simulink model "Microgrid_with_Utility_Connection"  (R2024b)
settings: Solver=daessc  StartTime=0.0  StopTime=inf  MaxStep=1e-3  RelTol=1e-3  AbsTol=1e-3
values from neighbouring files (symbols this model uses):
  Bat =     [initData.mat]
  droopFC1 = 0.05    [initData.mat]
  droopFC2 = 0.05    [initData.mat]
  droopP2 = 0.05    [initData.mat]
  droopQ1 = 0.05    [initData.mat]
  droopQ2 = 0.05    [initData.mat]
  Pref2 = 0.8    [initData.mat]
  Qref1 = 0    [initData.mat]
  Qref2 = 0    [initData.mat]
  timeACLoadCurtail = 200    [initData.mat]
  timeSolarCurtail = 200    [initData.mat]
  Ts = 5e-05    [initData.mat]
  Ts_AC = 0.0002    [initData.mat]
  Ts_DC = 0.001    [initData.mat]
  volt2 = [270.467186401 250.166401688 246.278575679 243.847178474 242.073246789 240.654489675 239.457734124 238.414696845 237.485238449 236.643553985 235.871256975 235.151075236 ... (161 elements, 1x161)]    [initData.mat]
undefined symbols (not defined in the file or in its folder): BattTempBp, CapLUTBp, CapSOCBp, DiscIntNeverNeededParam, Em, Np, Ns, RInt, Tc_Batt
libraries: nesl_utility x62, fl_lib x55, ee_lib x41, modbuslib x16, spsRMSLib x8, simulink x5, spsFourierLib x2, batteryecm_lib x1, eeTransforms x1
(part 2 of 3)

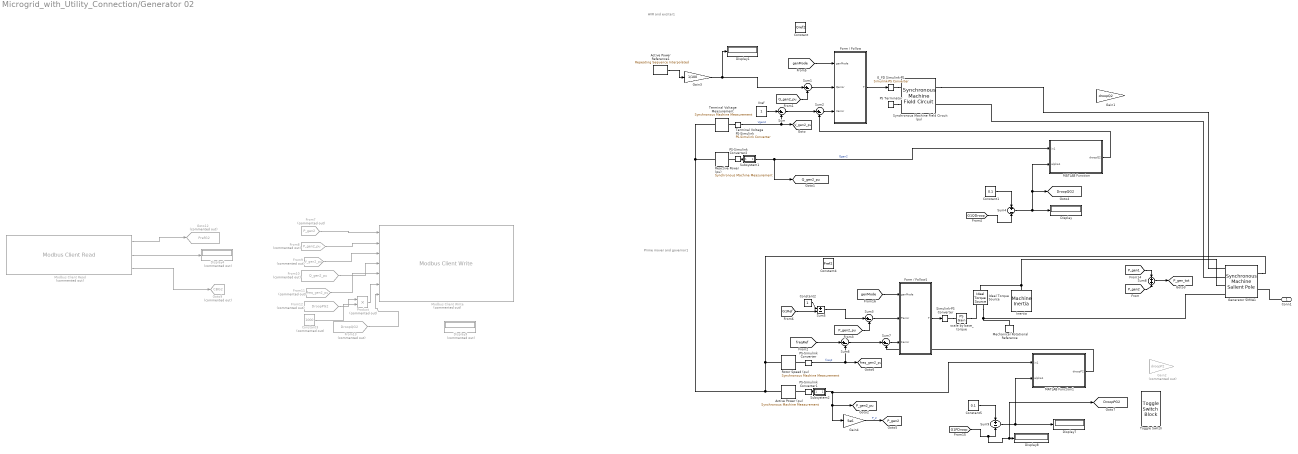
== system Microgrid_with_Utility_Connection/Generator 02 ==
  note: Prime mover
      | and governor1
  note: AVR and exciter1
  "Active Power (pu) " : ee_lib/Electromechanical/Synchronous/Synchronous Machine Measurement  output_idx=12
      settings: InternalSimscapePortConfiguration="{\"Bottom\":[],\"Left\":[{\"id\":\"pu_input\",\"label\":\"pu\",\"type\":\"input\"}],\"Right\":[{\"id\":\"pu_output\",\"label\":\"o\",\"type\":\"output\"}],\"Top\":[]}"
  Active Power Reference1 : simulink/Sources/Repeating Sequence Interpolated  OutValues=[0 0 0 0 0 0]  TimeValues=[100 110 120 130 140 500]  LookUpMeth=Interpolation-Use End Values  tsamp=Ts_AC  OutMin=[]  OutMax=[]  OutDataTypeStr=double  OutputDataTypeScalingMode=double  OutDataType=fixdt(0,8)  OutScaling=2^-10
  Constant : Constant  Value=Qref2
  Constant1 : Constant  Value=0.1
  Constant2 : Constant
  Constant3 : Constant  Commented=on  Value=1000
  Constant4 : Constant  Value=Pref2
  Constant5 : Constant  Value=0.1
  Display{,1,7..8} (4 alike) : Display
  Display4 : Display  Commented=on
      settings: Format=decimal (Stored Integer)  Decimation=4
  Display9 : Display  Commented=on
  "E_FD Simulink-PS " : nesl_utility/Simulink-PS Converter  PhysicalDomain=network_engine_domain  SubClassName=ps_input  LeftPortType=input  RightPortType=output  PseudoPeriodic=off  Frequencies=[]  NoiseDistribution=none  NoiseParameters=[]  Unit=1  AffineConversion=off  FilteringAndDerivatives=provide  SimscapeFilterOrder=1  InputFilterTimeConstant=.001  UdotUserProvided=0
  Form / Follow : Subsystem
  Form / Follow1 : Subsystem
  From10 : From  Commented=on  GotoTag=Q_gen2_pu  TagVisibility=global
  From11 : From  Commented=on  GotoTag=freq_gen2_pu  TagVisibility=global
  From12 : From  Commented=on  GotoTag=DroopPG2  TagVisibility=global
  From13 : From  Commented=on  GotoTag=DroopQG2  TagVisibility=global
  From7 : From  Commented=on  GotoTag=P_gen2  TagVisibility=global
  From8 : From  Commented=on  GotoTag=P_gen2_pu  TagVisibility=global
  From9 : From  Commented=on  GotoTag=V_gen2_pu  TagVisibility=global
  Gain1 : Gain  Gain=droopQ2
  Gain2 : Gain  Commented=on  Gain=droopP2
  Gain3 : Gain  Gain=1/100
  Gain4 : Gain  Gain=5e6
  Generator 5MVA1 : ee_lib/Electromechanical/Synchronous/Synchronous Machine Salient Pole  port_option=ee.enum.threePhasePort.composite  SRated=5e6 A*V  VRated=6600 V  FRated=50 Hz  nPolePairs=4  param_option=ee.enum.sm.parameterization.standard  fieldCircuitParameterization_option=ee.enum.sm.fieldparameterization.current  baseEfd=216.54 V  baseIfd=50 A  zero_sequence=ee.enum.park.zerosequence.exclude  axes_param=ee.enum.rotorangle.daxis  Ladu=0.9  Laqu=0.55  L0=0.15  Ll=0.15  Ra=0.011  Lfd=0.2571  Rfd=0.0006  L1d=0.2  R1d=0.0354  L1q=0.2567  R1q=0.0428  Xl=0.15  Xd=1.05  Xq=0.7  X0=0.15  Xdd=0.35  Xddd=0.25  Xqdd=0.325  d_option=ee.enum.circuit.open  Td0d=5.25 s  Tdd=1.75 s  Td0dd=0.03 s  Tddd=0.0214 s  q_option=ee.enum.circuit.open  Tq0dd=0.05 s  Tqdd=0.0232 s  saturation_option=ee.enum.saturation.exclude  saturation_ifd=[0.00, 0.48, 0.76, 1.38, 1.79]  saturation_Vag=[0.00, 0.43, 0.59, 0.71, 0.76]  initialization_option=ee.enum.sm.initialization.electrical  source_type=ee.enum.sm.load_flow_source_type.Swing  Vmag0=6600 V  Vang0=0 deg  Pt0=0.5 A*V  Qt0=0 A*V  minimum_pu=0.95  phase_search_range=[-inf, inf] deg  gmin=1e-6 S  connection_option=ee.enum.Connection.wye  num_q_dampers=1  rotor_offset=-pi / 2 rad  pu_psid_specify=on  pu_psid_priority=High  pu_psid=0  pu_psid_nominal_specify=off  pu_psid_nominal_value=1  pu_psid_nominal_unit=1  pu_psiq_specify=on  pu_psiq_priority=High  pu_psiq=0  pu_psiq_nominal_specify=off  pu_psiq_nominal_value=1  pu_psiq_nominal_unit=1  pu_psifd_specify=on  pu_psifd_priority=High  pu_psifd=0  pu_psifd_nominal_specify=off  pu_psifd_nominal_value=1  pu_psifd_nominal_unit=1  pu_psi1d_specify=on  pu_psi1d_priority=High  pu_psi1d=0  pu_psi1d_nominal_specify=off  pu_psi1d_nominal_value=1  pu_psi1d_nominal_unit=1  pu_psi1q_specify=on  pu_psi1q_priority=High  pu_psi1q=0  pu_psi1q_nominal_specify=off  pu_psi1q_nominal_value=1  pu_psi1q_nominal_unit=1  angular_position_diff_specify=on  angular_position_diff_priority=High  angular_position_diff=0 deg  angular_position_diff_nominal_specify=off  angular_position_diff_nominal_value=1  angular_position_diff_nominal_unit=deg  Tmeas=298.15 K  alpha=3.93e-3 1/K  stator_thermal_mass=100 J/K  rotor_thermal_mass=200 J/K  temperatureA_specify=off  temperatureA_priority=High  temperatureA=25 degC  temperatureA_nominal_specify=off  temperatureA_nominal_value=1  temperatureA_nominal_unit=degC  temperatureB_specify=off  temperatureB_priority=High  temperatureB=25 degC  temperatureB_nominal_specify=off  temperatureB_nominal_value=1  temperatureB_nominal_unit=degC  temperatureC_specify=off  temperatureC_priority=High  temperatureC=25 degC  temperatureC_nominal_specify=off  temperatureC_nominal_value=1  temperatureC_nominal_unit=degC  temperatureR_specify=off  temperatureR_priority=High  temperatureR=25 degC  temperatureR_nominal_specify=off  temperatureR_nominal_value=1  temperatureR_nominal_unit=degC
      settings: LogSimulationData=on  InternalSimscapePortConfiguration="{\"Bottom\":[],\"Left\":[{\"id\":\"fd_p\",\"label\":\"fd+\",\"type\":\"foundation.electrical.electrical\"},{\"id\":\"fd_n\",\"label\":\"fd-\",\"type\":\"foundation.electrical.electrical\"},{\"id\":\"R\",\"label\":\"R\",\"type\":\"foundation.mechanical.rotational.rotational\"},{\"id\":\"C\",\"label\":\"C\",\"type\":\"foundation.mechanical.rotational.rotational\"}],\"Right\":[{\"id\":\"pu_output\",\"label\":\"pu\",\"type\":\"output\"},{\"id\":\"N\",\"label\":\"~\",\"type\":\"foundation.electrical.three_phase\"}],\"Top\":[]}"
  Goto12 : Goto  Commented=on  GotoTag=PrefG2  TagVisibility=global
  Goto9 : Goto  Commented=on  GotoTag=CBG2  TagVisibility=global
  Ideal Torque Source : fl_lib/Mechanical/Mechanical Sources/Ideal Torque Source
  Inertia : ee_lib/Electromechanical/Mechanical/Machine Inertia  SRated=5e6 V*A  FRated=50 Hz  nPolePairs=4  inertia_option=2  J=27548 kg*m^2  H=3.525 s*W/V/A  damper_option=2  D=39.0509 N*m/(rad/s)  pu_D=0.01  initialization_option=2  fMechanical0=50 Hz  fElectrical0=50 Hz
      settings: LogSimulationData=on  InternalSimscapePortConfiguration="{\"Bottom\":[],\"Left\":[{\"id\":\"R\",\"label\":\"R\",\"type\":\"foundation.mechanical.rotational.rotational\"}],\"Right\":[],\"Top\":[]}"
  MATLAB Function : MATLAB Function  TreatAsAtomicUnit=on
  MATLAB Function1 : MATLAB Function  TreatAsAtomicUnit=on
  Mechanical Rotational Reference : fl_lib/Mechanical/Rotational Elements/Mechanical Rotational Reference
  Modbus Client Read : modbuslib/Modbus Client Read  Commented=on  RetainClient=gen2  ClientList=gen2  ConnectionEndpoint=192.168.1.203:502  ServerId=1  RegisterTable={ '1', 'PrefG2', '21', 'Holding Register', 'double', '1'; '2', 'QrefG2', '29', 'Holding Register', 'double', '1'; '3', 'CBG2', '38', 'Coil', 'bit', '1' }  SampleTime=1
  Modbus Client Write : modbuslib/Modbus Client Write  Commented=on  RetainClient=gen2  ClientList=gen2  ConnectionEndpoint=192.168.1.203:502  ServerId=1  RegisterTable={ '1', 'P_gen2', '1', 'Holding Register', 'double'; '2', 'P_gen2_pu', '5', 'Holding Register', 'double'; '3', 'V_gen2_pu', '9', 'Holding Register', 'double'; '4', 'Q_gen2_pu', '13', 'Holding Register', 'double'; '5', 'freq_gen2_pu', '17', 'Holding Register', 'double'; '6', 'DroopPG2', '25', 'Holding Register', 'double'; '7', 'DroopQG2', '34', 'Holding Register', 'double' }  SampleTime=1
  PS Terminator : fl_lib/Physical Signals/Sinks/PS Terminator
  PS-Simulink Converter : nesl_utility/PS-Simulink Converter  PhysicalDomain=network_engine_domain  SubClassName=ps_output  LeftPortType=input  RightPortType=output  PseudoPeriodic=off  Frequencies=[]  VectorFormat=1-D array  Unit=inherit  AffineConversion=off
  PS-Simulink Converter1 : nesl_utility/PS-Simulink Converter  PhysicalDomain=network_engine_domain  SubClassName=ps_output  LeftPortType=input  RightPortType=output  PseudoPeriodic=off  Frequencies=[]  VectorFormat=1-D array  Unit=inherit  AffineConversion=off
  PS-Simulink Converter2 : nesl_utility/PS-Simulink Converter  PhysicalDomain=network_engine_domain  SubClassName=ps_output  LeftPortType=input  RightPortType=output  PseudoPeriodic=off  Frequencies=[]  VectorFormat=1-D array  Unit=inherit  AffineConversion=off
  Product : Product  Commented=on
  Reactive Power (pu) : ee_lib/Electromechanical/Synchronous/Synchronous Machine Measurement  output_idx=13
      settings: InternalSimscapePortConfiguration="{\"Bottom\":[],\"Left\":[{\"id\":\"pu_input\",\"label\":\"pu\",\"type\":\"input\"}],\"Right\":[{\"id\":\"pu_output\",\"label\":\"o\",\"type\":\"output\"}],\"Top\":[]}"
  Rotor Speed (pu) : ee_lib/Electromechanical/Synchronous/Synchronous Machine Measurement  output_idx=4
      settings: InternalSimscapePortConfiguration="{\"Bottom\":[],\"Left\":[{\"id\":\"pu_input\",\"label\":\"pu\",\"type\":\"input\"}],\"Right\":[{\"id\":\"pu_output\",\"label\":\"o\",\"type\":\"output\"}],\"Top\":[]}"
  Simulink-PS Converter : nesl_utility/Simulink-PS Converter  PhysicalDomain=network_engine_domain  SubClassName=ps_input  LeftPortType=input  RightPortType=output  PseudoPeriodic=off  Frequencies=[]  NoiseDistribution=none  NoiseParameters=[]  Unit=1  AffineConversion=off  FilteringAndDerivatives=provide  SimscapeFilterOrder=1  InputFilterTimeConstant=0.001  UdotUserProvided=0
  Subsystem1 : Subsystem
  Subsystem2 : Subsystem
  Sum{,1..3,6..7} (6 alike) : Sum  Inputs=|+-
  Sum4 : Sum  Inputs=+-
  Sum5 : Sum  Inputs=+-
  Sum8 : Sum
  Sum9 : Sum  Inputs=+-
  Synchronous Machine Field Circuit (pu) : ee_lib/Electromechanical/Synchronous/Synchronous Machine Field Circuit  unit_option=ee.enum.unit.pu  SRated=5e6 V*A  FRated=50 Hz  fieldCircuitParameterization_option=2  baseEfd=92.95 V  baseIfd=50 A  parameterization_option=2  Ladu=1.66  Rfd=0.0006  Xl=0.15  Xd=1.05  Xdd=0.35  Xddd=0.23  d_option=ee.enum.circuit.open  Td0d=5.25 s  Tdd=1.3260 s  Td0dd=0.03 s  Tddd=0.0230 s
      settings: LogSimulationData=on  InternalSimscapePortConfiguration="{\"Bottom\":[],\"Left\":[{\"id\":\"Efd_pu\",\"label\":\"Efd_pu\",\"type\":\"input\"},{\"id\":\"Ifd_pu\",\"label\":\"Ifd_pu\",\"type\":\"output\"}],\"Right\":[{\"id\":\"fd_p\",\"label\":\"fd+\",\"type\":\"foundation.electrical.electrical\"},{\"id\":\"fd_n\",\"label\":\"fd-\",\"type\":\"foundation.electrical.electrical\"}],\"Top\":[]}"
  Terminal Voltage Measurement : ee_lib/Electromechanical/Synchronous/Synchronous Machine Measurement  output_idx=14
      settings: LogSimulationData=on  InternalSimscapePortConfiguration="{\"Bottom\":[],\"Left\":[{\"id\":\"pu_input\",\"label\":\"pu\",\"type\":\"input\"}],\"Right\":[{\"id\":\"pu_output\",\"label\":\"o\",\"type\":\"output\"}],\"Top\":[]}"
  Terminal Voltage PS-Simulink : nesl_utility/PS-Simulink Converter  PhysicalDomain=network_engine_domain  SubClassName=ps_output  LeftPortType=input  RightPortType=output  PseudoPeriodic=off  Frequencies=[]  VectorFormat=1-D array  Unit=1  AffineConversion=off
  Toggle Switch : ToggleSwitchBlock
      settings: Values={{'Off', 'On'}, [0 0.05]}
  Vref : Constant  SampleTime=Ts_AC
  scale by base_torque : fl_lib/Physical Signals/Functions/PS Gain  gain=53051.6 N*m
  Conn1 : PMIOPort  Side=Right
  tag scope: DroopPG2=global, DroopQG2=global, P_gen2=global, P_gen2_pu=global, P_gen_tot=global, Q_gen2_pu=global, V_gen2_pu=global, freq_gen2_pu=global
  wires:
  Gain3/1 -> Sum1/1, Display1/1
  Active Power Reference1/1 -> Gain3/1
  MATLAB Function/1(droopQ2) -> Sum2/2
  [G1QDroop] -> Sum4/2
  Constant1/1 -> Sum4/1
  Sum4/1 -> [DroopQG2], MATLAB Function/2(alpha1), Display/1
  Form / Follow/1(T) -> "E_FD Simulink-PS "/1
  Sum2/1 -> Form / Follow/3(Verror)
  [genMode] -> Form / Follow/1(genMode)
  Sum1/1 -> Form / Follow/2(Qerror)
  [Q_gen2_pu] -> Sum1/2
  Subsystem1/1(in1) -> MATLAB Function/1(in1), [Q_gen2_pu]  "Qgen2"
  Vref/1 -> Sum/1
  Sum/1 -> Sum2/1
  Terminal Voltage PS-Simulink/1 -> [V_gen2_pu], Sum/2  "Vgen2"
  PS-Simulink Converter2/1 -> Subsystem1/1(In1)
  Constant3/1 -> Product/2
  Product/1 -> Modbus Client Write/6
  From12/1 -> Product/1
  From13/1 -> Modbus Client Write/7
  From11/1 -> Modbus Client Write/5
  From10/1 -> Modbus Client Write/4
  From9/1 -> Modbus Client Write/3
  From8/1 -> Modbus Client Write/2
  Modbus Client Read/3 -> Goto9/1
  From7/1 -> Modbus Client Write/1
  Modbus Client Read/2 -> Display4/1
  Sum5/1 -> Sum3/1
  [G1Ref] -> Sum5/2
  Constant2/1 -> Sum5/1
  [G1PDroop] -> [DroopPG2], Display8/1, Sum9/2
  Constant5/1 -> Sum9/1
  Sum9/1 -> MATLAB Function1/2(alpha1), Display7/1
  Subsystem2/1(in) -> MATLAB Function1/1(in1), [P_gen2_pu], Gain4/1
  Form / Follow1/1(T) -> Simulink-PS Converter/1
  Sum7/1 -> Form / Follow1/3(Ferror)
  Sum3/1 -> Form / Follow1/2(Perror)
  [genMode] -> Form / Follow1/1(genMode)
  [P_gen2_pu] -> Sum3/2
  Sum8/1 -> [P_gen_tot]
  [P_gen2] -> Sum8/2
  [P_gen1] -> Sum8/1
  Gain4/1 -> [P_gen2]  "P_2"
  PS-Simulink Converter1/1 -> Subsystem2/1(In1)
  PS-Simulink Converter/1 -> [freq_gen2_pu], Sum6/2  "freq2"
  [freqRef] -> Sum6/1
  Sum6/1 -> Sum7/1
  MATLAB Function1/1(droopP2) -> Sum7/2
  Modbus Client Read/1 -> Goto12/1
  connections:
  Ideal Torque Source/RConn2 -- Mechanical Rotational Reference/LConn1 -- Generator 5MVA1/LConn4
  Inertia/LConn1 -- Generator 5MVA1/LConn3 -- Ideal Torque Source/LConn1
  Conn1/RConn1 -- Generator 5MVA1/RConn2
  Synchronous Machine Field Circuit (pu)/RConn1 -- Generator 5MVA1/LConn1
  Generator 5MVA1/LConn2 -- Synchronous Machine Field Circuit (pu)/RConn2
  PS Terminator/LConn1 -- Synchronous Machine Field Circuit (pu)/LConn2
  "E_FD Simulink-PS "/RConn1 -- Synchronous Machine Field Circuit (pu)/LConn1
  "Active Power (pu) "/LConn1 -- Reactive Power (pu)/LConn1 -- Terminal Voltage Measurement/LConn1 -- Generator 5MVA1/RConn1 -- Rotor Speed (pu)/LConn1
  Terminal Voltage Measurement/RConn1 -- Terminal Voltage PS-Simulink/LConn1
  PS-Simulink Converter2/LConn1 -- Reactive Power (pu)/RConn1
  Simulink-PS Converter/RConn1 -- scale by base_torque/LConn1
  scale by base_torque/RConn1 -- Ideal Torque Source/RConn1
  PS-Simulink Converter/LConn1 -- Rotor Speed (pu)/RConn1
  PS-Simulink Converter1/LConn1 -- "Active Power (pu) "/RConn1

== system Microgrid_with_Utility_Connection/Grid Synchronization ==
  note: breaker command: 1 - islanded (PCC open)
      | 0 - connect to utility (PCC closed)
  note: 1 - start sycnhronisation
      | 0 - stay islanded
  note: microgrid frequency (pu)
  note: utility grid phase angle
  note: microgrid phase angle
  note: new frequency reference sent to
      | microgrid governer
  note: utility grid frequency (pu)
  note: frequency step size (how aggressive we tune frequency)
  Constant1 : Constant  Value=1e-5
  Constant2 : Constant
  Grid Synchronization1 : MATLAB Function  TreatAsAtomicUnit=on
  Unit Delay : UnitDelay  InitialCondition=1  SampleTime=Ts_AC  HasFrameUpgradeWarning=on
  Unit Delay1 : UnitDelay  InitialCondition=1  SampleTime=Ts_AC  HasFrameUpgradeWarning=on
  tag scope: freqRef=global, gridEnable=global
  wires:
  Grid Synchronization1/2(gridEnable) -> Unit Delay/1  "gridEnable"
  Constant1/1 -> Grid Synchronization1/1(deltaF)
  [phiMicro] -> Grid Synchronization1/5(phiMicro)
  Unit Delay1/1 -> [freqRef]
  [freq_gen1_pu] -> Grid Synchronization1/3(freqMicro)
  Grid Synchronization1/1(freqRef) -> Unit Delay1/1
  Constant2/1 -> Grid Synchronization1/2(freqUtility)
  Unit Delay/1 -> [gridEnable]
  [phiUtility] -> Grid Synchronization1/4(phiUtility)
  [synchStart] -> Grid Synchronization1/6(synchStart)

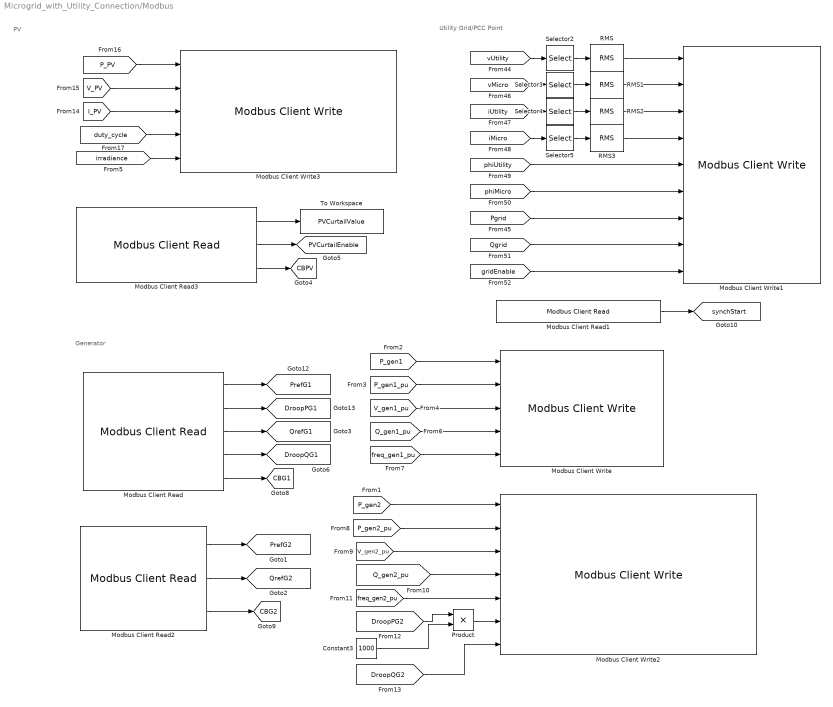
== system Microgrid_with_Utility_Connection/Modbus ==
  note: PV
  note: Utility Grid/PCC Point
  note: Generator
  Constant3 : Constant  Value=1000
  Modbus Client Read : modbuslib/Modbus Client Read  RetainClient=gen1  ClientList=gen1  ConnectionEndpoint=192.168.1.202:502  ServerId=1  RegisterTable={ '1', 'PrefG1', '21', 'Holding Register', 'double', '1'; '2', 'DroopPG1', '25', 'Holding Register', 'double', '1'; '3', 'QrefG1', '29', 'Holding Register', 'double', '1'; '4', 'DroopQG1', '34', 'Holding Register', 'double', '1'; '5', 'CBG1', '38', 'Coil', 'bit', '1' }  SampleTime=1
  Modbus Client Read1 : modbuslib/Modbus Client Read  RetainClient=ModbusClient  ClientList=ModbusClient  ConnectionEndpoint=192.168.1.201:502  ServerId=1  RegisterTable={ '1', 'synchStart', '38', 'Coil', 'bit', '1' }  SampleTime=1
  Modbus Client Read2 : modbuslib/Modbus Client Read  RetainClient=gen2  ClientList=gen2  ConnectionEndpoint=192.168.1.203:502  ServerId=1  RegisterTable={ '1', 'PrefG2', '21', 'Holding Register', 'double', '1'; '2', 'QrefG2', '29', 'Holding Register', 'double', '1'; '3', 'CBG2', '38', 'Coil', 'bit', '1' }  SampleTime=1
  Modbus Client Read3 : modbuslib/Modbus Client Read  RetainClient=pv  ClientList=pv  ConnectionEndpoint=192.168.1.204:502  ServerId=1  RegisterTable={ '1', 'PvCurtailValue', '21', 'Holding Register', 'double', '1'; '2', 'curtail enable', '25', 'Coil', 'bit', '1'; '3', 'CBPV', '29', 'Coil', 'bit', '1' }  SampleTime=1
  Modbus Client Write : modbuslib/Modbus Client Write  RetainClient=gen1  ClientList=gen1  ConnectionEndpoint=192.168.1.202:502  ServerId=1  RegisterTable={ '1', 'P_gen1', '1', 'Holding Register', 'double'; '2', 'P_gen1_pu', '5', 'Holding Register', 'double'; '3', 'V_gen1_pu', '9', 'Holding Register', 'double'; '4', 'Q_gen1_pu', '13', 'Holding Register', 'double'; '5', 'freq_gen1_pu', '17', 'Holding Register', 'double' }  SampleTime=1
  Modbus Client Write1 : modbuslib/Modbus Client Write  RetainClient=ModbusClient  ClientList=ModbusClient  ConnectionEndpoint=192.168.1.201:502  ServerId=1  RegisterTable={ '1', 'vUtility_rms', '1', 'Holding Register', 'double'; '2', 'vMicro_rms', '5', 'Holding Register', 'double'; '3', 'iUtility_rms', '9', 'Holding Register', 'double'; '4', 'iMicro_rms', '13', 'Holding Register', 'double'; '5', 'phiUtility', '17', 'Holding Register', 'double'; '6', 'phiMicro', '21', 'Holding Register', 'double'; '7', 'Pgrid', '25', 'Holding Register', 'double'; '8', 'Qgrid', '29', 'Holding Register', 'double'; '9', 'gridEnable', '34', 'Coil', 'bit' }  SampleTime=1
  Modbus Client Write2 : modbuslib/Modbus Client Write  RetainClient=gen2  ClientList=gen2  ConnectionEndpoint=192.168.1.203:502  ServerId=1  RegisterTable={ '1', 'P_gen2', '1', 'Holding Register', 'double'; '2', 'P_gen2_pu', '5', 'Holding Register', 'double'; '3', 'V_gen2_pu', '9', 'Holding Register', 'double'; '4', 'Q_gen2_pu', '13', 'Holding Register', 'double'; '5', 'freq_gen2_pu', '17', 'Holding Register', 'double'; '6', 'DroopPG2', '25', 'Holding Register', 'double'; '7', 'DroopQG2', '34', 'Holding Register', 'double' }  SampleTime=1
  Modbus Client Write3 : modbuslib/Modbus Client Write  RetainClient=pv  ClientList=pv  ConnectionEndpoint=192.168.1.204:502  ServerId=1  RegisterTable={ '1', 'P_PV', '1', 'Holding Register', 'double'; '2', 'V_PV', '5', 'Holding Register', 'double'; '3', 'I_PV', '9', 'Holding Register', 'double'; '4', 'duty cycle', '13', 'Holding Register', 'double'; '5', 'irradiance', '17', 'Holding Register', 'double' }  SampleTime=1
  Product : Product
  RMS{,1..3} (4 alike) : spsRMSLib/RMS  TrueRMS=on  Freq=50  RMSInit=120  Ts=0
  Selector{2..5} (4 alike) : Selector  InputPortWidth=3  IndexOptions=Index vector (dialog)  Indices=1  OutputSizes=1
  To Workspace : ToWorkspace  VariableName=PVCurtailValue  SaveFormat=Timeseries  SampleTime=-1
  tag scope: CBG1=global, CBG2=global, CBPV=global, DroopPG1=global, DroopQG1=global, PVCurtailEnable=global, PrefG1=global, PrefG2=global, QrefG1=global, QrefG2=global, synchStart=global
  wires:
  [V_gen1_pu] -> Modbus Client Write/3
  [P_gen1_pu] -> Modbus Client Write/2
  Modbus Client Read/1 -> [PrefG1]
  [P_gen1] -> Modbus Client Write/1
  [freq_gen1_pu] -> Modbus Client Write/5
  [Q_gen1_pu] -> Modbus Client Write/4
  Modbus Client Read/2 -> [DroopPG1]
  Modbus Client Read/5 -> [CBG1]
  [iMicro] -> Selector5/1
  RMS2/1 -> Modbus Client Write1/3
  RMS/1 -> Modbus Client Write1/1
  RMS3/1 -> Modbus Client Write1/4
  [iUtility] -> Selector4/1
  [phiUtility] -> Modbus Client Write1/5
  [Qgrid] -> Modbus Client Write1/8
  [Pgrid] -> Modbus Client Write1/7
  Selector4/1 -> RMS2/1
  Selector5/1 -> RMS3/1
  RMS1/1 -> Modbus Client Write1/2
  Modbus Client Read1/1 -> [synchStart]
  [vMicro] -> Selector3/1
  [vUtility] -> Selector2/1
  [phiMicro] -> Modbus Client Write1/6
  [gridEnable] -> Modbus Client Write1/9
  Selector2/1 -> RMS/1
  Selector3/1 -> RMS1/1
  Constant3/1 -> Product/2
  [P_gen2] -> Modbus Client Write2/1
  [DroopPG2] -> Product/1
  [V_gen2_pu] -> Modbus Client Write2/3
  Product/1 -> Modbus Client Write2/6
  Modbus Client Read2/3 -> [CBG2]
  Modbus Client Read2/2 -> [QrefG2]
  [DroopQG2] -> Modbus Client Write2/7
  [freq_gen2_pu] -> Modbus Client Write2/5
  [Q_gen2_pu] -> Modbus Client Write2/4
  [P_gen2_pu] -> Modbus Client Write2/2
  Modbus Client Read2/1 -> [PrefG2]
  Modbus Client Read3/3 -> [CBPV]
  [P_PV] -> Modbus Client Write3/1
  Modbus Client Read3/1 -> To Workspace/1
  [irradiance] -> Modbus Client Write3/5
  [duty_cycle] -> Modbus Client Write3/4
  [I_PV] -> Modbus Client Write3/3
  Modbus Client Read3/2 -> [PVCurtailEnable]
  [V_PV] -> Modbus Client Write3/2
  Modbus Client Read/3 -> [QrefG1]
  Modbus Client Read/4 -> [DroopQG1]

== system Microgrid_with_Utility_Connection/PQ meas ==
  PS-Simulink Converter : nesl_utility/PS-Simulink Converter  PhysicalDomain=network_engine_domain  SubClassName=ps_output  LeftPortType=input  RightPortType=output  PseudoPeriodic=off  Frequencies=[]  VectorFormat=1-D array  Unit=W  AffineConversion=off
  PS-Simulink Converter1 : nesl_utility/PS-Simulink Converter  PhysicalDomain=network_engine_domain  SubClassName=ps_output  LeftPortType=input  RightPortType=output  PseudoPeriodic=off  Frequencies=[]  VectorFormat=1-D array  Unit=V*A  AffineConversion=off
  Power Sensor (Three-Phase) : ee_lib/Sensors & Transducers/Power Sensor (Three-Phase)  load_type=ee.enum.passive.type_balanced.balanced  f0=50 Hz
      settings: InternalSimscapePortConfiguration="{\"Bottom\":[],\"Left\":[{\"id\":\"N1\",\"label\":\"~1\",\"type\":\"foundation.electrical.three_phase\"}],\"Right\":[{\"id\":\"N2\",\"label\":\"~2\",\"type\":\"foundation.electrical.three_phase\"}],\"Top\":[{\"id\":\"Pm\",\"label\":\"P\",\"type\":\"output\"},{\"id\":\"Qm\",\"label\":\"Q\",\"type\":\"output\"}]}"
  Subsystem : Subsystem
  Subsystem1 : Subsystem
  ~1 : PMIOPort  Side=Left
  ~2 : PMIOPort  Port=2  Side=Right
  tag scope: P_load=global, Q_load=global
  wires:
  PS-Simulink Converter1/1 -> Subsystem1/1(In1)
  Subsystem1/1(Out1) -> [Q_load]  "Q_load"
  Subsystem/1(Out1) -> [P_load]  "P_load"
  PS-Simulink Converter/1 -> Subsystem/1(In1)
  connections:
  ~2/RConn1 -- Power Sensor (Three-Phase)/RConn1
  Power Sensor (Three-Phase)/LConn1 -- ~1/RConn1
  PS-Simulink Converter/LConn1 -- Power Sensor (Three-Phase)/LConn2
  PS-Simulink Converter1/LConn1 -- Power Sensor (Three-Phase)/LConn3

== system Microgrid_with_Utility_Connection/PV Array ==
  Display : Display
  ERef : fl_lib/Electrical/Electrical Elements/Electrical Reference
  Product1 : Product
  Repeating Sequence Interpolated : simulink/Sources/Repeating Sequence Interpolated  OutValues=[1e-3 1e-3 1 1]*1000  TimeValues=[0 1 5 300]  LookUpMeth=Interpolation-Use End Values  tsamp=Ts_DC  OutMin=[]  OutMax=[]  OutDataTypeStr=double  OutputDataTypeScalingMode=double  OutDataType=fixdt(0,8)  OutScaling=2^-10
  Sensing Current : Subsystem
      settings: PortSchema="{\"entries\":[{\"content\":{\"sides\":[{\"content\":{\"connectorIds\":[\"LConn1\"]},\"type\":\"ConnectorPlacement.EquallySpacedRectSide\",\"uuid\":\"08eaf192-3836-4d70-9f6a-c3aee0977ea6\"},{\"content\":{\"connectorIds\":[\"RConn1\"],\"side\":\"RIGHT\"},\"type\":\"ConnectorPlacement.EquallySpacedRectSide\",\"uuid\":\"69615d36-c1bf-4d31-b3e4-77c73286e7c7\"},{\"content\":{\"connectorIds\":[\"Out1\"],\"side\":\"TOP\"},\"type\":\"ConnectorPlacement.EquallySpacedRectSide\",\"uuid\":\"21e31d90-f675-47e5-98f5-1bf7e6a5fdbe\"}]},\"type\":\"ConnectorPlacement.EquallySpacedConnector\",\"uuid\":\"068abd2e-abc9-41d7-b40e-d83d3e3b9346\"}],\"packageUris\":[\"http://schema.mathworks.com/mf0/Connector/R2020b\"],\"version\":\"1.0\"}"
      mask Display: disp('i')
  Simulink-PS Converter : nesl_utility/Simulink-PS Converter  PhysicalDomain=network_engine_domain  SubClassName=ps_input  LeftPortType=input  RightPortType=output  PseudoPeriodic=off  Frequencies=[]  NoiseDistribution=none  NoiseParameters=[]  Unit=1  AffineConversion=off  FilteringAndDerivatives=provide  SimscapeFilterOrder=1  InputFilterTimeConstant=0.001  UdotUserProvided=0
  Solar Cell : ee_lib/Sources/Solar Cell  PartSpecification="{\"DatasetId\":\"Amerisolar|AS_6M30_HC_320W|simscape.electrical.solarCell\",\"DisplayName\":\"Amerisolar:AS_6M30_HC_320W\"}"  prm=3  Isc=10.14 A  Voc=0.67 V  Is=3.24823447983853e-07 A  Is2=9.37081970792037e-10 A  Iph=10.140005507508 A  Ir0=1000 W/m^2  ec=1.51118472243322  N2=2.60259908345858  Rs=1.94548269975201e-05 Ohm  Rp=682.95993142779 Ohm  N_series=60*100  N_parallel=30  TIPH1=0.000499942933005141 1/K  EG=1.12 eV  TXIS1=4.23641510120988  TXIS2=16.2689137700667  TRS1=0.243341028305912  TRP1=0 % Parameter not set  Tmeas=25 degC  TFIXED=30 degC  thermal_mass=100 % Parameter not set J/K  initial_temperature=25 degC
      settings: AttributesFormatString=Amerisolar:AS_6M30_HC_320W
  Terminator : Terminator
  sensing voltage : Subsystem
      settings: PortSchema="{\"entries\":[{\"content\":{\"sides\":[{\"content\":{\"connectorIds\":[\"LConn1\"]},\"type\":\"ConnectorPlacement.EquallySpacedRectSide\",\"uuid\":\"08eaf192-3836-4d70-9f6a-c3aee0977ea6\"},{\"content\":{\"connectorIds\":[\"RConn1\"],\"side\":\"RIGHT\"},\"type\":\"ConnectorPlacement.EquallySpacedRectSide\",\"uuid\":\"69615d36-c1bf-4d31-b3e4-77c73286e7c7\"},{\"content\":{\"connectorIds\":[],\"side\":\"TOP\"},\"type\":\"ConnectorPlacement.EquallySpacedRectSide\",\"uuid\":\"21e31d90-f675-47e5-98f5-1bf7e6a5fdbe\"},{\"content\":{\"connectorIds\":[\"Out1\"],\"side\":\"BOTTOM\"},\"type\":\"ConnectorPlacement.EquallySpacedRectSide\",\"uuid\":\"23a77980-6beb-4147-b48e-adf9e1983263\"}]},\"type\":\"ConnectorPlacement.EquallySpacedConnector\",\"uuid\":\"068abd2e-abc9-41d7-b40e-d83d3e3b9346\"}],\"packageUris\":[\"http://schema.mathworks.com/mf0/Connector/R2020b\"],\"version\":\"1.0\"}"
      mask Display: disp('v')
  - : PMIOPort  Side=Left
  -1 : PMIOPort  Port=2  Side=Left
  tag scope: I_PV=global, V_PV=global, irradiance=global
  wires:
  sensing voltage/1(V) -> Display/1, [V_PV], Product1/2  "V_PV"
  Product1/1 -> Terminator/1  "P_PV"
  Repeating Sequence Interpolated/1 -> [irradiance], Simulink-PS Converter/1  "irradiance"
  Sensing Current/1(I) -> [I_PV], Product1/1  "I_PV"
  connections:
  Solar Cell/LConn1 -- Simulink-PS Converter/RConn1
  Solar Cell/LConn2 -- Sensing Current/LConn1
  sensing voltage/RConn1 -- Solar Cell/RConn1 -- ERef/LConn1 -- -1/RConn1
  sensing voltage/LConn1 -- -/RConn1 -- Sensing Current/RConn1

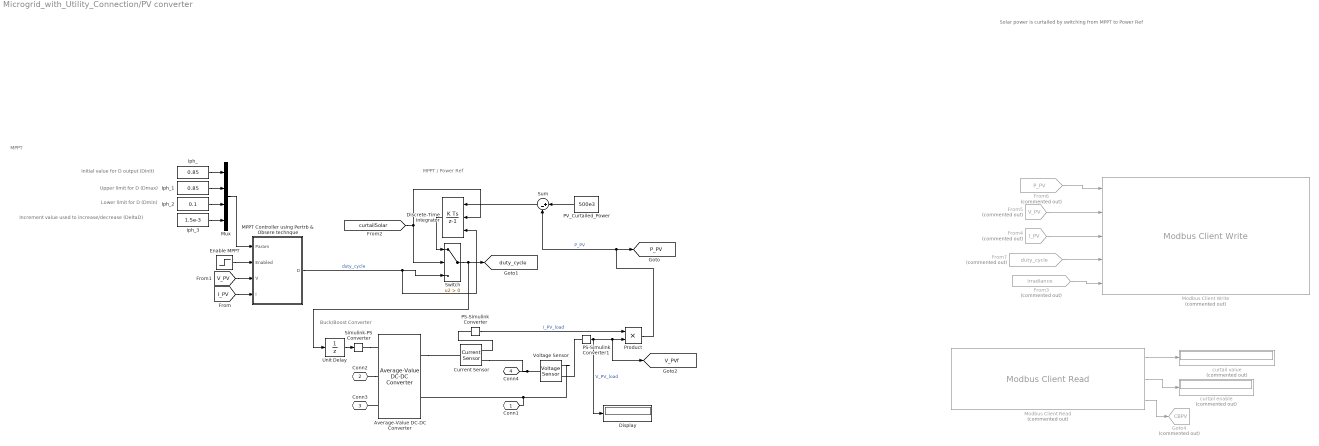
== system Microgrid_with_Utility_Connection/PV converter ==
  note: Lower limit for D (Dmin)
  note: Upper limit for D (Dmax)
  note: Increment value used to increase/decrease (DeltaD)
  note: Initial value for D output (Dinit)
  note: Solar power is curtailed by switching from MPPT to Power Ref
  note: MPPT / Power Ref
  note: MPPT
  note: Buck/Boost Converter
  Average-Value DC-DC Converter : ee_lib/Semiconductors & Converters/Converters/Average-Value DC-DC Converter  control_option=ee.enum.converters.controlinput.dutycycle  converter_type=ee.enum.converters.dcdctype.buckboost  efficiency_option=ee.enum.converters.efficiency.constant  efficiency_fixed=100  i_vec=[0, 2, 5] A  efficiency_vec=[90, 95, 98]
      settings: InternalSimscapePortConfiguration="{\"Bottom\":[],\"Left\":[{\"id\":\"DutyCycle\",\"label\":\"DutyCycle\",\"type\":\"input\"},{\"id\":\"p1\",\"label\":\"1+\",\"type\":\"foundation.electrical.electrical\"},{\"id\":\"n1\",\"label\":\"1-\",\"type\":\"foundation.electrical.electrical\"}],\"Right\":[{\"id\":\"p2\",\"label\":\"2+\",\"type\":\"foundation.electrical.electrical\"},{\"id\":\"n2\",\"label\":\"2-\",\"type\":\"foundation.electrical.electrical\"}],\"Top\":[]}"
  Current Sensor : fl_lib/Electrical/Electrical Sensors/Current Sensor
  Discrete-Time Integrator : DiscreteIntegrator  gainval=1e-6  ExternalReset=rising  InitialConditionSource=external  SampleTime=-1  ICPrevOutput=DiscIntNeverNeededParam  ICPrevScaledInput=DiscIntNeverNeededParam
  Display : Display
  Enable MPPT : Step  Time=0.1  SampleTime=Ts_DC
  From3 : From  Commented=on  GotoTag=irradiance  TagVisibility=global
  From4 : From  Commented=on  GotoTag=I_PV  TagVisibility=global
  From5 : From  Commented=on  GotoTag=V_PV  TagVisibility=global
  From6 : From  Commented=on  GotoTag=P_PV  TagVisibility=global
  From7 : From  Commented=on  GotoTag=duty_cycle  TagVisibility=global
  Goto4 : Goto  Commented=on  GotoTag=CBPV  TagVisibility=global
  Iph_ : Constant  Value=0.85  SampleTime=Ts_DC
  Iph_1 : Constant  Value=0.85  SampleTime=Ts_DC
  Iph_2 : Constant  Value=0.1  SampleTime=Ts_DC
  Iph_3 : Constant  Value=1.5e-3  SampleTime=Ts_DC
  "MPPT Controller using Pertrb & Obsere technque " : MATLAB Function  SystemSampleTime=Ts
  Modbus Client Read : modbuslib/Modbus Client Read  Commented=on  RetainClient=pv  ClientList=pv  ConnectionEndpoint=192.168.1.204:502  ServerId=1  RegisterTable={ '1', 'PvCurtailValue', '21', 'Holding Register', 'double', '1'; '2', 'curtail enable', '25', 'Coil', 'bit', '1'; '3', 'CBPV', '29', 'Coil', 'bit', '1' }  SampleTime=1
  Modbus Client Write : modbuslib/Modbus Client Write  Commented=on  RetainClient=pv  ClientList=pv  ConnectionEndpoint=192.168.1.204:502  ServerId=1  RegisterTable={ '1', 'P_PV', '1', 'Holding Register', 'double'; '2', 'V_PV', '5', 'Holding Register', 'double'; '3', 'I_PV', '9', 'Holding Register', 'double'; '4', 'duty cycle', '13', 'Holding Register', 'double'; '5', 'irradiance', '17', 'Holding Register', 'double' }  SampleTime=1
  Mux : Mux
  PS-Simulink Converter : nesl_utility/PS-Simulink Converter  PhysicalDomain=network_engine_domain  SubClassName=ps_output  LeftPortType=input  RightPortType=output  PseudoPeriodic=off  Frequencies=[]  VectorFormat=1-D array  Unit=inherit  AffineConversion=off
  PS-Simulink Converter1 : nesl_utility/PS-Simulink Converter  PhysicalDomain=network_engine_domain  SubClassName=ps_output  LeftPortType=input  RightPortType=output  PseudoPeriodic=off  Frequencies=[]  VectorFormat=1-D array  Unit=inherit  AffineConversion=off
  PV_Curtailed_Power : Constant  Value=500e3
  Product : Product
  Simulink-PS Converter : nesl_utility/Simulink-PS Converter  PhysicalDomain=network_engine_domain  SubClassName=ps_input  LeftPortType=input  RightPortType=output  PseudoPeriodic=off  Frequencies=[]  NoiseDistribution=none  NoiseParameters=[]  Unit=1  AffineConversion=off  FilteringAndDerivatives=provide  SimscapeFilterOrder=1  InputFilterTimeConstant=0.001  UdotUserProvided=0
  Sum : Sum  Inputs=|+-
  Switch : Switch  Criteria=u2 > Threshold  SaturateOnIntegerOverflow=off  InputSameDT=off
  Unit Delay : UnitDelay  InitialCondition=0.99  SampleTime=-1  HasFrameUpgradeWarning=on
  Voltage Sensor : fl_lib/Electrical/Electrical Sensors/Voltage Sensor
  curtail enable : Display  Commented=on
      settings: Format=decimal (Stored Integer)  Decimation=4
  curtail value : Display  Commented=on
      settings: Format=decimal (Stored Integer)  Decimation=4
  Conn1 : PMIOPort  Side=Left
  Conn2 : PMIOPort  Port=2  Side=Left
  Conn3 : PMIOPort  Port=3  Side=Left
  Conn4 : PMIOPort  Port=4  Side=Left
  tag scope: P_PV=global, V_PVf=global, duty_cycle=global
  wires:
  From7/1 -> Modbus Client Write/4
  Enable MPPT/1 -> "MPPT Controller using Pertrb & Obsere technque "/2(Enabled)
  Modbus Client Read/2 -> curtail enable/1
  Iph_1/1 -> Mux/2
  Mux/1 -> "MPPT Controller using Pertrb & Obsere technque "/1(Param)
  [V_PV] -> "MPPT Controller using Pertrb & Obsere technque "/3(V)
  Unit Delay/1 -> Simulink-PS Converter/1
  From4/1 -> Modbus Client Write/3
  Iph_2/1 -> Mux/3
  PS-Simulink Converter1/1 -> Display/1, [V_PVf], Product/2  "V_PV_load"
  [curtailSolar] -> Discrete-Time Integrator/2, Switch/2
  Iph_/1 -> Mux/1
  From5/1 -> Modbus Client Write/2
  PS-Simulink Converter/1 -> Product/1  "I_PV_load"
  Iph_3/1 -> Mux/4
  From6/1 -> Modbus Client Write/1
  Sum/1 -> Discrete-Time Integrator/1
  Modbus Client Read/3 -> Goto4/1
  "MPPT Controller using Pertrb & Obsere technque "/1(D) -> Discrete-Time Integrator/3, Switch/3  "duty_cycle"
  PV_Curtailed_Power/1 -> Sum/1
  Modbus Client Read/1 -> curtail value/1
  Product/1 -> Sum/2, [P_PV]  "P_PV"
  From3/1 -> Modbus Client Write/5
  [I_PV] -> "MPPT Controller using Pertrb & Obsere technque "/4(I)
  Discrete-Time Integrator/1 -> Switch/1
  Switch/1 -> Unit Delay/1, [duty_cycle]
  connections:
  Conn2/RConn1 -- Average-Value DC-DC Converter/LConn2
  Current Sensor/RConn2 -- Voltage Sensor/LConn1 -- Conn4/RConn1
  Simulink-PS Converter/RConn1 -- Average-Value DC-DC Converter/LConn1
  Average-Value DC-DC Converter/RConn1 -- Current Sensor/LConn1
  Voltage Sensor/RConn2 -- Conn1/RConn1 -- Average-Value DC-DC Converter/RConn2
  PS-Simulink Converter/LConn1 -- Current Sensor/RConn1
  Average-Value DC-DC Converter/LConn3 -- Conn3/RConn1
  PS-Simulink Converter1/LConn1 -- Voltage Sensor/RConn1

== system Microgrid_with_Utility_Connection/Power Converter ==
  AC/DC Power Conversion : Subsystem
      settings: PortSchema="{\"entries\":[{\"content\":{\"sides\":[{\"content\":{\"connectorIds\":[\"LConn1\"]},\"type\":\"ConnectorPlacement.EquallySpacedRectSide\",\"uuid\":\"019ca52f-1b20-4f8a-8000-26047d27ba44\"},{\"content\":{\"connectorIds\":[\"RConn1\",\"RConn2\"],\"side\":\"RIGHT\"},\"type\":\"ConnectorPlacement.EquallySpacedRectSide\",\"uuid\":\"bc0710a3-2fa6-4c07-a357-204360cbd971\"},{\"content\":{\"connectorIds\":[\"In1\",\"In2\"],\"side\":\"TOP\"},\"type\":\"ConnectorPlacement.EquallySpacedRectSide\",\"uuid\":\"62c22250-eba7-4d66-a03a-98d0551949f6\"}]},\"type\":\"ConnectorPlacement.EquallySpacedConnector\",\"uuid\":\"4a6536c9-62d3-4a93-9f4d-cdcce83d66f7\"}],\"packageUris\":[\"http://schema.mathworks.com/mf0/Connector/R2020b\"],\"version\":\"1.0\"}"
      mask Display: disp('Ideal AC/DC\nPower Conversion')
  Current Sensor : fl_lib/Electrical/Electrical Sensors/Current Sensor
  Display : Display
  Electrical Reference : fl_lib/Electrical/Electrical Elements/Electrical Reference
  PS-Simulink Converter : nesl_utility/PS-Simulink Converter  PhysicalDomain=network_engine_domain  SubClassName=ps_output  LeftPortType=input  RightPortType=output  PseudoPeriodic=off  Frequencies=[]  VectorFormat=inherit  Unit=inherit  AffineConversion=off
  PS-Simulink Converter1 : nesl_utility/PS-Simulink Converter  PhysicalDomain=network_engine_domain  SubClassName=ps_output  LeftPortType=input  RightPortType=output  PseudoPeriodic=off  Frequencies=[]  VectorFormat=inherit  Unit=inherit  AffineConversion=off
  Product : Product
  Qref : simulink/Sources/Repeating Sequence Interpolated  OutValues=[0 0 0 0]*1e5  TimeValues=[0 11 13 50]  LookUpMeth=Interpolation-Use End Values  tsamp=Ts_AC  OutMin=[]  OutMax=[]  OutDataTypeStr=double  OutputDataTypeScalingMode=double  OutDataType=fixdt(0,8)  OutScaling=2^-10
  Solver Configuration : nesl_utility/Solver Configuration  PhysicalDomain=network_engine_domain  SubClassName=solver  LeftPortType=input  RightPortType=generic  Tones=[]  Harmonics=[]  SimulateNoise=off  Profile=off  UseLocalSampling=off  EnableSwitchedLinearOptims=on  FrequencyDomain=off  UseCCode=off  RelTol=0.001  AbsTol=1e-06  MinStep=1e-09  ToWorkspace=off  RevertToSquareIcSolve=off  NumHomotopyIterations=100  PhasorMode=off  PhasorModeNumHarmonics=1  ConsistencySolver=NEWTON_FTOL  IndexReductionMethod=DerivativeReplacement  DoDC=off  ResidualTolerance=1e-09  ConsistencyTolSource=GLOBAL  ConsistencyAbsTol=0.001  ConsistencyRelTol=0.001  ConsistencyTolFactor=0.001  UseLocalSolver=on  LocalSolverChoice=NE_PARTITIONING_ADVANCER  ResolveIndetEquations=on  FunctionEvalNumThread=1  LocalSolverSampleTime=Ts_DC  DoFixedCost=on  MaxNonlinIter=1  MaxModeIter=2  ComputeImpulses=off  ImpulseIterations=2  LinearAlgebra=auto  LinearAlgebraNumThread=0  EquationFormulation=NE_TIME_EF  DelaysMemoryBudget=1024  AutomaticFiltering=on  FilteringTimeConstant=0.001  PartitionStorageMethod=AS_NEEDED  PartitionMemoryBudget=1024  PartitionMethod=ROBUST  MultibodyUseLocalSolver=off  MultibodyLocalSolverChoice=ODE1  MultibodyLocalSolverSampleTime=0.001
  Voltage Sensor : fl_lib/Electrical/Electrical Sensors/Voltage Sensor
  ~ : PMIOPort  Side=Left
  + : PMIOPort  Port=2  Side=Right
  - : PMIOPort  Port=3  Side=Right
  wires:
  Qref/1 -> AC/DC Power Conversion/2(Qref)
  [P_AC_ref] -> AC/DC Power Conversion/1(Pref)
  PS-Simulink Converter1/1 -> Product/2
  PS-Simulink Converter/1 -> Product/1
  Product/1 -> Display/1
  connections:
  AC/DC Power Conversion/LConn1 -- ~/RConn1
  Current Sensor/LConn1 -- Voltage Sensor/LConn1 -- AC/DC Power Conversion/RConn1
  AC/DC Power Conversion/RConn2 -- -/RConn1 -- Voltage Sensor/RConn2 -- Electrical Reference/LConn1
  Solver Configuration/RConn1 -- +/RConn1 -- Current Sensor/RConn2
  PS-Simulink Converter/LConn1 -- Current Sensor/RConn1
  PS-Simulink Converter1/LConn1 -- Voltage Sensor/RConn1

== system Microgrid_with_Utility_Connection/Reactive Power Load ==
  Electrical Reference1 : fl_lib/Electrical/Electrical Elements/Electrical Reference
  PS Divide : fl_lib/Physical Signals/Functions/PS Divide
  PS Product : fl_lib/Physical Signals/Functions/PS Product
  Phase Splitter1 : ee_lib/Connectors & References/Phase Splitter
  Reactive Power Reference : simulink/Sources/Repeating Sequence Interpolated  OutValues=[1e-6 1e-6 1e-6]*6e6*2*pi*50  TimeValues=[0 1 50]  LookUpMeth=Interpolation-Use End Values  tsamp=Ts_AC  OutMin=[]  OutMax=[]  OutDataTypeStr=double  OutputDataTypeScalingMode=double  OutDataType=fixdt(0,8)  OutScaling=2^-10
  Simulink-PS Converter1 : nesl_utility/Simulink-PS Converter  PhysicalDomain=network_engine_domain  SubClassName=ps_input  LeftPortType=input  RightPortType=output  PseudoPeriodic=off  Frequencies=[]  NoiseDistribution=none  NoiseParameters=[]  Unit=V*A*rad/s  AffineConversion=off  FilteringAndDerivatives=provide  SimscapeFilterOrder=1  InputFilterTimeConstant=0.001  UdotUserProvided=0
  Variable Inductor : ee_lib/Passive/Variable Inductor  prm=2  Lmin=1e-6 H  g=0 1/Ohm  i0=0 A  phi0=0 Wb
      settings: InternalSimscapePortConfiguration="{\"Bottom\":[],\"Left\":[{\"id\":\"L\",\"label\":\"L\",\"type\":\"input\"},{\"id\":\"p\",\"label\":\"+\",\"type\":\"foundation.electrical.electrical\"}],\"Right\":[{\"id\":\"n\",\"label\":\"-\",\"type\":\"foundation.electrical.electrical\"}],\"Top\":[]}"
  Variable Inductor1 : ee_lib/Passive/Variable Inductor  prm=2  Lmin=1e-6 H  g=0 1/Ohm  i0=0 A  phi0=0 Wb
      settings: InternalSimscapePortConfiguration="{\"Bottom\":[],\"Left\":[{\"id\":\"L\",\"label\":\"L\",\"type\":\"input\"},{\"id\":\"p\",\"label\":\"+\",\"type\":\"foundation.electrical.electrical\"}],\"Right\":[{\"id\":\"n\",\"label\":\"-\",\"type\":\"foundation.electrical.electrical\"}],\"Top\":[]}"
  Variable Inductor2 : ee_lib/Passive/Variable Inductor  prm=2  Lmin=1e-6 H  g=0 1/Ohm  i0=0 A  phi0=0 Wb
      settings: InternalSimscapePortConfiguration="{\"Bottom\":[],\"Left\":[{\"id\":\"L\",\"label\":\"L\",\"type\":\"input\"},{\"id\":\"p\",\"label\":\"+\",\"type\":\"foundation.electrical.electrical\"}],\"Right\":[{\"id\":\"n\",\"label\":\"-\",\"type\":\"foundation.electrical.electrical\"}],\"Top\":[]}"
  Vnom : fl_lib/Physical Signals/Sources/PS Constant  constant=6600*0.98 V
  Conn1 : PMIOPort  Side=Left
  wires:
  Reactive Power Reference/1 -> Simulink-PS Converter1/1
  connections:
  Phase Splitter1/RConn3 -- Variable Inductor2/LConn2
  PS Product/LConn2 -- PS Product/LConn1 -- Vnom/RConn1
  PS Divide/LConn1 -- PS Product/RConn1
  Simulink-PS Converter1/RConn1 -- PS Divide/LConn2
  Variable Inductor/LConn1 -- Variable Inductor2/LConn1 -- Variable Inductor1/LConn1 -- PS Divide/RConn1
  Variable Inductor1/LConn2 -- Phase Splitter1/RConn2
  Variable Inductor/RConn1 -- Variable Inductor1/RConn1 -- Variable Inductor2/RConn1 -- Electrical Reference1/LConn1
  Phase Splitter1/RConn1 -- Variable Inductor/LConn2
  Phase Splitter1/LConn1 -- Conn1/RConn1

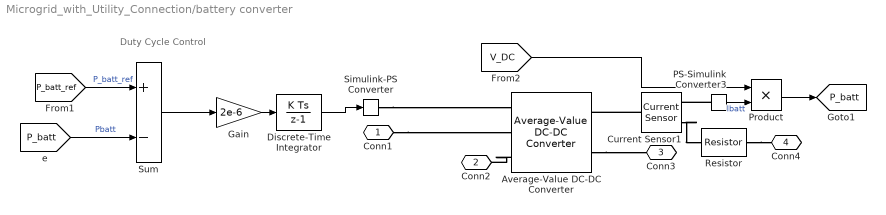
== system Microgrid_with_Utility_Connection/battery converter ==
  note: Duty Cycle Control
  Average-Value DC-DC Converter : ee_lib/Semiconductors & Converters/Converters/Average-Value DC-DC Converter  control_option=ee.enum.converters.controlinput.dutycycle  converter_type=ee.enum.converters.dcdctype.buckboost  efficiency_option=ee.enum.converters.efficiency.constant  efficiency_fixed=100  i_vec=[0, 2, 5] A  efficiency_vec=[90, 95, 98]
      settings: InternalSimscapePortConfiguration="{\"Bottom\":[],\"Left\":[{\"id\":\"DutyCycle\",\"label\":\"DutyCycle\",\"type\":\"input\"},{\"id\":\"p1\",\"label\":\"1+\",\"type\":\"foundation.electrical.electrical\"},{\"id\":\"n1\",\"label\":\"1-\",\"type\":\"foundation.electrical.electrical\"}],\"Right\":[{\"id\":\"p2\",\"label\":\"2+\",\"type\":\"foundation.electrical.electrical\"},{\"id\":\"n2\",\"label\":\"2-\",\"type\":\"foundation.electrical.electrical\"}],\"Top\":[]}"
  Current Sensor1 : fl_lib/Electrical/Electrical Sensors/Current Sensor
  Discrete-Time Integrator : DiscreteIntegrator  InitialCondition=0.5  SampleTime=Ts_DC  LimitOutput=on  UpperSaturationLimit=0.99  LowerSaturationLimit=0  ICPrevOutput=DiscIntNeverNeededParam  ICPrevScaledInput=DiscIntNeverNeededParam
  Gain : Gain  Gain=2e-6
  PS-Simulink Converter3 : nesl_utility/PS-Simulink Converter  PhysicalDomain=network_engine_domain  SubClassName=ps_output  LeftPortType=input  RightPortType=output  PseudoPeriodic=off  Frequencies=[]  VectorFormat=1-D array  Unit=inherit  AffineConversion=off
  Product : Product
  Resistor : fl_lib/Electrical/Electrical Elements/Resistor  R=1e-3 Ohm  i_specify=off  i_priority=None  i=0 A  i_nominal_specify=off  i_nominal_value=1  i_nominal_unit=A  v_specify=off  v_priority=None  v=0 V  v_nominal_specify=off  v_nominal_value=1  v_nominal_unit=V
  Simulink-PS Converter : nesl_utility/Simulink-PS Converter  PhysicalDomain=network_engine_domain  SubClassName=ps_input  LeftPortType=input  RightPortType=output  PseudoPeriodic=off  Frequencies=[]  NoiseDistribution=none  NoiseParameters=[]  Unit=1  AffineConversion=off  FilteringAndDerivatives=provide  SimscapeFilterOrder=1  InputFilterTimeConstant=0.001  UdotUserProvided=0
  Sum : Sum  Inputs=+-
  Conn1 : PMIOPort  Side=Left
  Conn2 : PMIOPort  Port=2  Side=Left
  Conn3 : PMIOPort  Port=3  Side=Right
  Conn4 : PMIOPort  Port=4  Side=Right
  tag scope: P_batt=global
  wires:
  PS-Simulink Converter3/1 -> Product/2  "Ibatt"
  Discrete-Time Integrator/1 -> Simulink-PS Converter/1
  Product/1 -> [P_batt]
  [P_batt] -> Sum/2  "Pbatt"
  [V_DC] -> Product/1
  [P_batt_ref] -> Sum/1  "P_batt_ref"
  Gain/1 -> Discrete-Time Integrator/1
  Sum/1 -> Gain/1
  connections:
  Average-Value DC-DC Converter/LConn3 -- Conn2/RConn1
  Current Sensor1/RConn2 -- Resistor/LConn1
  Conn1/RConn1 -- Average-Value DC-DC Converter/LConn2
  PS-Simulink Converter3/LConn1 -- Current Sensor1/RConn1
  Current Sensor1/LConn1 -- Average-Value DC-DC Converter/RConn1
  Simulink-PS Converter/RConn1 -- Average-Value DC-DC Converter/LConn1
  Resistor/RConn1 -- Conn4/RConn1
  Average-Value DC-DC Converter/RConn2 -- Conn3/RConn1
